simulink model "TourismusdynamikSimConstant"  (R2022b)
settings: Solver=VariableStepAuto  StartTime=0.0  StopTime=timeFinal  MaxStep=timeStep  RelTol=1e-3
values from neighbouring files (symbols this model uses):
  pKapazitaet = iParaSets(j).pKapazitaet    [Tourismusdynamik.m]
  pRegenerationsZeit = iParaSets(j).pRegenerationsZeit    [Tourismusdynamik.m]
  pUmsatzanteilFuerUmwelt = iParaSets(j).pUmsatzanteilFuerUmwelt    [Tourismusdynamik.m]
  pVerbesserungsRate = iParaSets(j).pVerbesserungsRate    [Tourismusdynamik.m]
  pVerbrauchsRate = iParaSets(j).pVerbrauchsRate    [Tourismusdynamik.m]
  pVerlustRate = iParaSets(j).pVerlustRate    [Tourismusdynamik.m]
  pWerbeEinfluss = iParaSets(j).pWerbeEinfluss    [Tourismusdynamik.m]
settings Model: Creator=benja  LastModifiedBy=benja

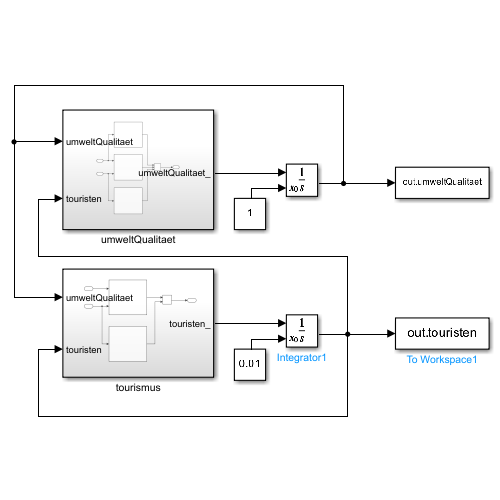
[thumbnail: Simulink's stored preview of the top-level diagram]
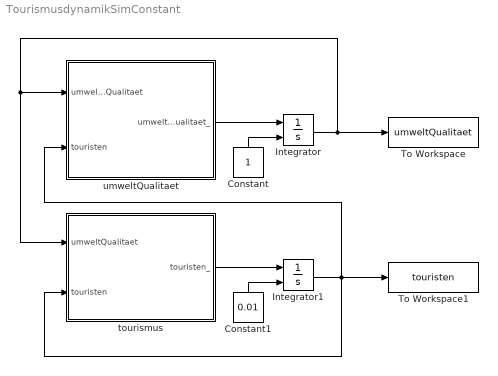
== system TourismusdynamikSimConstant ==
  Constant : Constant
  Constant1 : Constant  Value=0.01
  Integrator : Integrator  InitialConditionSource=external  InitialCondition=1
  Integrator1 : Integrator  InitialConditionSource=external  InitialCondition=0.1
  To Workspace : ToWorkspace  VariableName=umweltQualitaet  SaveFormat=Timeseries  SampleTime=-1
  To Workspace1 : ToWorkspace  VariableName=touristen  SaveFormat=Timeseries  SampleTime=-1
  tourismus : Subsystem
  umweltQualitaet : Subsystem
  wires:
  umweltQualitaet/1(umweltQualitaet_) -> Integrator/1
  tourismus/1(touristen_) -> Integrator1/1
  Integrator1/1 -> umweltQualitaet/2(touristen), To Workspace1/1, tourismus/2(touristen)
  Integrator/1 -> umweltQualitaet/1(umweltQualitaet), tourismus/1(umweltQualitaet), To Workspace/1
  Constant/1 -> Integrator/2
  Constant1/1 -> Integrator1/2

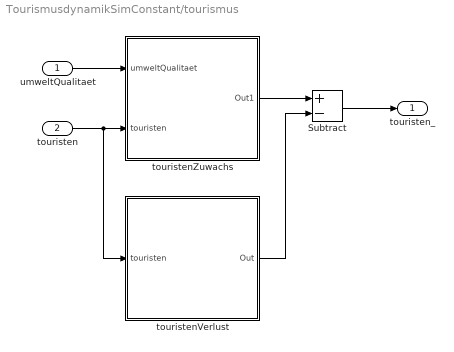
== system TourismusdynamikSimConstant/tourismus ==
  umweltQualitaet : Inport
  touristen : Inport  Port=2
  Subtract : Sum  Inputs=+-
  touristenVerlust : Subsystem
  touristenZuwachs : Subsystem
  touristen_ : Outport
  wires:
  touristen/1 -> touristenVerlust/1(touristen), touristenZuwachs/2(touristen)
  umweltQualitaet/1 -> touristenZuwachs/1(umweltQualitaet)
  touristenZuwachs/1(Out1) -> Subtract/1
  touristenVerlust/1(Out) -> Subtract/2
  Subtract/1 -> touristen_/1

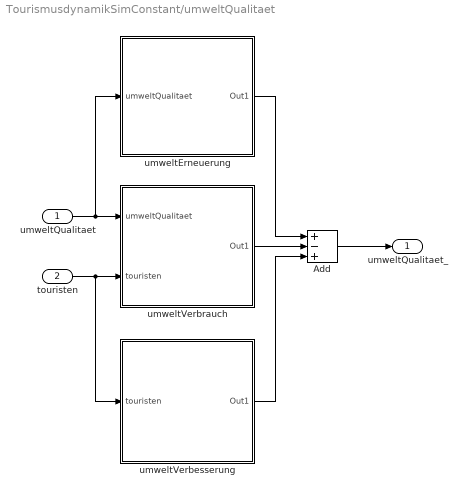
== system TourismusdynamikSimConstant/umweltQualitaet ==
  umweltQualitaet : Inport
  touristen : Inport  Port=2
  Add : Sum  Inputs=+-+
  umweltErneuerung : Subsystem
  umweltVerbesserung : Subsystem
  umweltVerbrauch : Subsystem
  umweltQualitaet_ : Outport
  wires:
  umweltQualitaet/1 -> umweltErneuerung/1(umweltQualitaet), umweltVerbrauch/1(umweltQualitaet)
  touristen/1 -> umweltVerbesserung/1(touristen), umweltVerbrauch/2(touristen)
  umweltErneuerung/1(Out1) -> Add/1
  umweltVerbrauch/1(Out1) -> Add/2
  umweltVerbesserung/1(Out1) -> Add/3
  Add/1 -> umweltQualitaet_/1

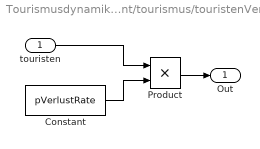
== system TourismusdynamikSimConstant/tourismus/touristenVerlust ==
  touristen : Inport
  Constant : Constant  Value=pVerlustRate
  Product : Product
  Out : Outport
  wires:
  touristen/1 -> Product/1
  Constant/1 -> Product/2
  Product/1 -> Out/1

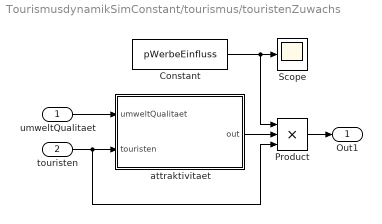
== system TourismusdynamikSimConstant/tourismus/touristenZuwachs ==
  umweltQualitaet : Inport
  touristen : Inport  Port=2
  Constant : Constant  Value=pWerbeEinfluss
  Product : Product  Inputs=3
  Scope : Scope
  attraktivitaet : Subsystem
  Out1 : Outport
  wires:
  umweltQualitaet/1 -> attraktivitaet/1(umweltQualitaet)
  touristen/1 -> Product/3, attraktivitaet/2(touristen)
  attraktivitaet/1(out) -> Product/2
  Product/1 -> Out1/1
  Constant/1 -> Scope/1, Product/1

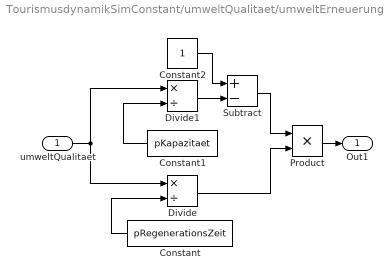
== system TourismusdynamikSimConstant/umweltQualitaet/umweltErneuerung ==
  umweltQualitaet : Inport
  Constant : Constant  Value=pRegenerationsZeit
  Constant1 : Constant  Value=pKapazitaet
  Constant2 : Constant
  Divide : Product  Inputs=*/
  Divide1 : Product  Inputs=*/
  Product : Product
  Subtract : Sum  Inputs=+-
  Out1 : Outport
  wires:
  umweltQualitaet/1 -> Divide/1, Divide1/1
  Constant/1 -> Divide/2
  Divide1/1 -> Subtract/2
  Constant1/1 -> Divide1/2
  Constant2/1 -> Subtract/1
  Subtract/1 -> Product/1
  Divide/1 -> Product/2
  Product/1 -> Out1/1

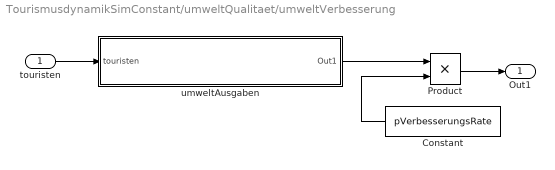
== system TourismusdynamikSimConstant/umweltQualitaet/umweltVerbesserung ==
  touristen : Inport
  Constant : Constant  Value=pVerbesserungsRate
  Product : Product
  umweltAusgaben : Subsystem
  Out1 : Outport
  wires:
  touristen/1 -> umweltAusgaben/1(touristen)
  Product/1 -> Out1/1
  umweltAusgaben/1(Out1) -> Product/1
  Constant/1 -> Product/2

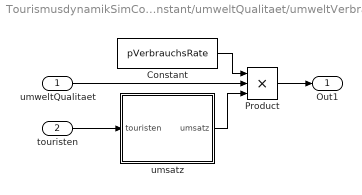
== system TourismusdynamikSimConstant/umweltQualitaet/umweltVerbrauch ==
  umweltQualitaet : Inport
  touristen : Inport  Port=2
  Constant : Constant  Value=pVerbrauchsRate
  Product : Product  Inputs=3
  umsatz : Subsystem
  Out1 : Outport
  wires:
  touristen/1 -> umsatz/1(touristen)
  Constant/1 -> Product/1
  umweltQualitaet/1 -> Product/2
  umsatz/1(umsatz) -> Product/3
  Product/1 -> Out1/1

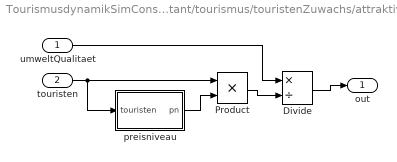
== system TourismusdynamikSimConstant/tourismus/touristenZuwachs/attraktivitaet ==
  umweltQualitaet : Inport
  touristen : Inport  Port=2
  Divide : Product  Inputs=*/
  Product : Product
  preisniveau : Subsystem
  out : Outport
  wires:
  touristen/1 -> preisniveau/1(touristen), Product/1
  Divide/1 -> out/1
  preisniveau/1(pn) -> Product/2
  Product/1 -> Divide/2
  umweltQualitaet/1 -> Divide/1

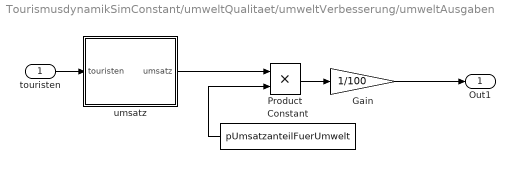
== system TourismusdynamikSimConstant/umweltQualitaet/umweltVerbesserung/umweltAusgaben ==
  touristen : Inport
  Constant : Constant  Value=pUmsatzanteilFuerUmwelt
  Gain : Gain  Gain=1/100
  Product : Product
  umsatz : Subsystem
  Out1 : Outport
  wires:
  touristen/1 -> umsatz/1(touristen)
  umsatz/1(umsatz) -> Product/1
  Constant/1 -> Product/2
  Gain/1 -> Out1/1
  Product/1 -> Gain/1

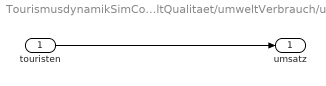
== system TourismusdynamikSimConstant/umweltQualitaet/umweltVerbrauch/umsatz ==
  touristen : Inport
  umsatz : Outport
  wires:
  touristen/1 -> umsatz/1

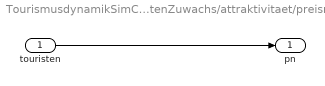
== system TourismusdynamikSimConstant/tourismus/touristenZuwachs/attraktivitaet/preisniveau ==
  touristen : Inport
  pn : Outport
  wires:
  touristen/1 -> pn/1

== system TourismusdynamikSimConstant/umweltQualitaet/umweltVerbesserung/umweltAusgaben/umsatz ==
  touristen : Inport
  umsatz : Outport
  wires:
  touristen/1 -> umsatz/1
